simulink model "Parte2"  (R2025b)
settings: Solver=VariableStepAuto  StartTime=0.0  StopTime=3  MaxStep=0.01  RelTol=1e-3
settings Model: Creator=Nehir RT  LastModifiedBy=Nehir RT

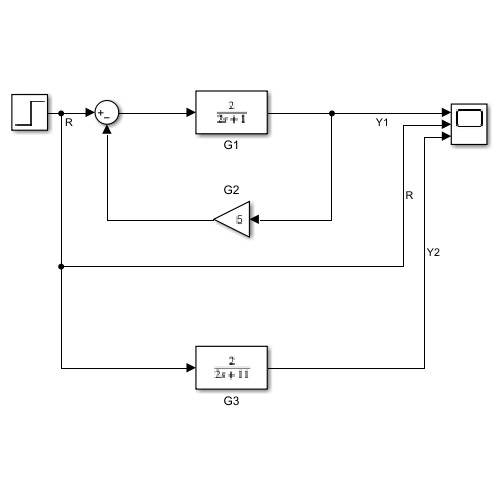
[thumbnail: Simulink's stored preview of the top-level diagram]
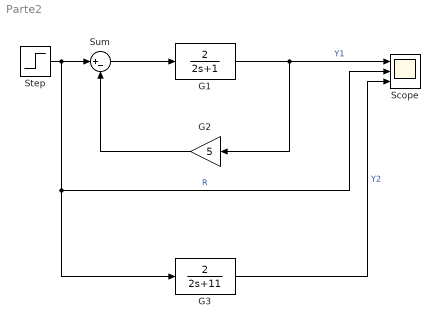
== system Parte2 ==
  G1 : TransferFcn  Numerator=[2]  Denominator=[2 1]
  G2 : Gain  Gain=5
  G3 : TransferFcn  Numerator=[2]  Denominator=[2 11]
  Scope : Scope  NumInputPorts=3
      settings: ActiveDisplayYMinimum=-0.031875110569237308  ActiveDisplayYMaximum=0.45023900660782906
  Step : Step  SampleTime=0
  Sum : Sum  Inputs=|+-
  wires:
  Sum/1 -> G1/1
  Step/1 -> Scope/2, G3/1, Sum/1  "R"
  G1/1 -> G2/1, Scope/1  "Y1"
  G2/1 -> Sum/2
  G3/1 -> Scope/3  "Y2"
